simulink model "Aufgabe2_2"  (Simulink 9.1)
settings: Solver=VariableStepAuto  StartTime=0.0  StopTime=10.0  RelTol=1e-3
InitFcn:
  | run('Auf2_1_Initialisierung.m') % Initialisierung
values from neighbouring files (symbols this model uses):
  H = inv(A)*(phi-eye(3))*B    [Aufgabe2_2_linmod.m]
  phi = expm(h*A)    [Aufgabe2_2_linmod.m]
undefined symbols (not defined in the file or in its folder): C, D
libraries: cstblocks x1
settings Model: Creator=kleist  LastModifiedBy=kleist
settings DataIOCC: SaveFormat=Dataset
settings OptimizationCC: LifeSpan=auto
settings DebuggingCC: UnderspecifiedInitializationDetection=Simplified  MergeDetectMultiDrivingBlocksExec=error  SFUnexpectedBacktrackingDiag=error  SFNoUnconditionalDefaultTransitionDiag=error  SFExecutionAtInitializationDiag=warning
settings HardwareCC: ProdBitPerPointer=64  ProdBitPerSizeT=64  ProdBitPerPtrDiffT=64  ProdLargestAtomicFloat=Float  ProdIntDivRoundTo=Zero  ProdEndianess=LittleEndian  ProdWordSize=64  ProdHWDeviceType=Intel->x86-64 (Windows64)
settings ModelReferenceCC: PropagateSignalLabelsOutOfModel=on
settings CodeAppCC: StateflowObjectComments=off
settings GRTTargetCC: TargetLangStandard=C99 (ISO)  CombineOutputUpdateFcns=on  GRTInterface=off
settings ConfigComp: CovMetricSettings=dwe  CovHtmlReporting=off  CovSaveCumulativeToWorkspaceVar=off  CovSaveSingleToWorkspaceVar=off  CovExternalEMLEnable=on

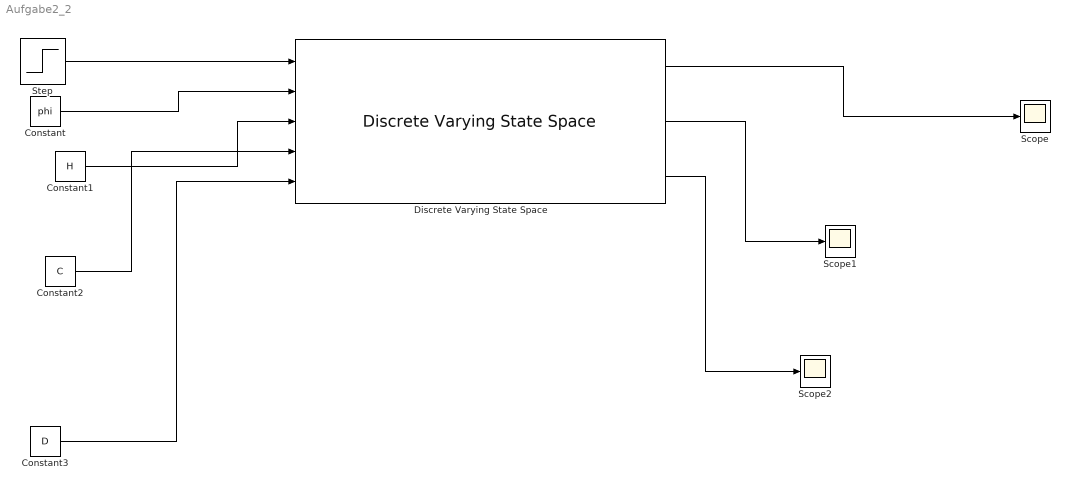
== system Aufgabe2_2 ==
  Constant : Constant  Value=phi  VectorParams1D=off
  Constant1 : Constant  Value=H  VectorParams1D=off
  Constant2 : Constant  Value=C  VectorParams1D=off
  Constant3 : Constant  Value=D  VectorParams1D=off
  Discrete Varying State Space : cstblocks/Linear Parameter Varying/Discrete Varying State Space  x0=[0;0;0]  Ts=0.015  OutputX=on  OutputDX=on
      settings: SourceProductName=Control System Toolbox  SourceProductBaseCode=CT
  Scope : Scope
  Scope1 : Scope
  Scope2 : Scope
  Step : Step  Time=0  SampleTime=0
  wires:
  Step/1 -> Discrete Varying State Space/1
  Constant/1 -> Discrete Varying State Space/2
  Constant1/1 -> Discrete Varying State Space/3
  Constant2/1 -> Discrete Varying State Space/4
  Constant3/1 -> Discrete Varying State Space/5
  Discrete Varying State Space/1 -> Scope/1
  Discrete Varying State Space/2 -> Scope1/1
  Discrete Varying State Space/3 -> Scope2/1
